simulink library "simCryogenics_lib"  (R2016a)
settings: Solver=VariableStepAuto  StartTime=0.0  StopTime=10.0  RelTol=1e-3
undefined symbols (not defined in the file or in its folder): gcbh, simscape
(part 2 of 4)

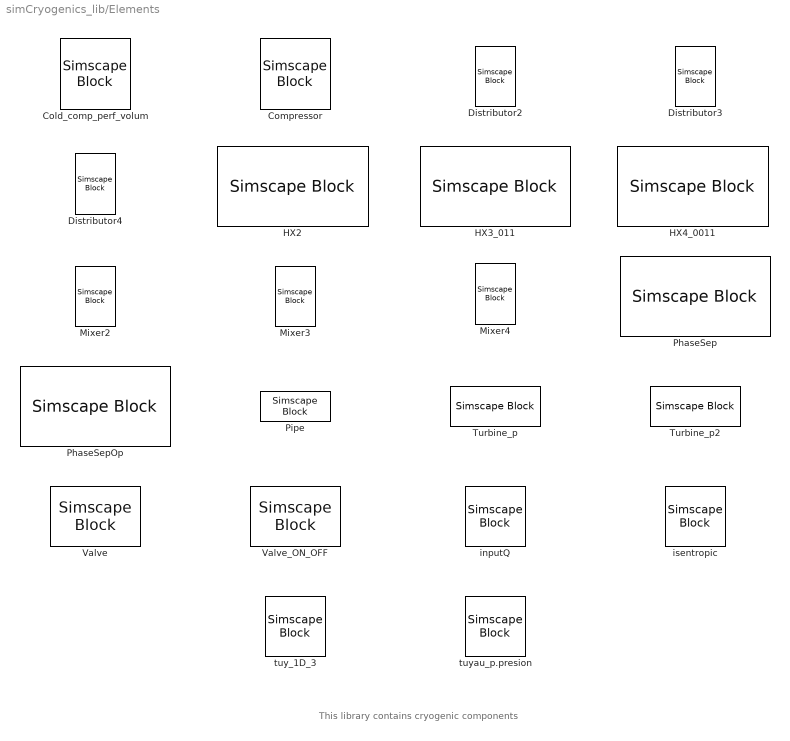
== system simCryogenics_lib/Elements ==
  note: This library contains cryogenic components
  Cold_comp_perf_volum : SimscapeBlock  DialogController=NetworkEngine.DynNeDlgSource  LoadFcn=simscape.compiler.sli.internal.callback('LoadFcn',gcbh);  SourceFile=simCryogenics.Elements.Cold_comp_perf_volum  mask(Cold_comp_perf_volum){ComponentPath=simCryogenics.Elements.Cold_comp_perf_volum, ComponentVariants=simCryogenics.Elements.Cold_comp_perf_volum, ComponentVariantNames=Cold_comp_perf_volum, ClassName=Cold_comp_perf_volum, SchemaVersion=1, rho0=1, rho0_unit=kg/m^3, rho0_conf=compiletime, eta=0.9, eta_unit=1, eta_conf=compiletime, vol=1, vol_unit=1, vol_conf=compiletime, Sin_specify=off, Sin_priority=None, Sin=0, Sin_unit=kJ/kg, HoutIs_specify=off, HoutIs_priority=None, HoutIs=0, HoutIs_unit=kJ/kg, rho_specify=off, rho_priority=None, rho=1, rho_unit=kg/m^3}
      mask prompts: rho0 "Nominal inlet density"; eta "Nominal efficiency"; vol "Volumetric"; Sin_specify "Sin"; Sin_priority "Sin"; HoutIs_specify "HoutIs"; HoutIs_priority "HoutIs"; rho_specify "rho"; rho_priority "rho"
      mask help:
      | This component is a perfect Cold Compressor with constant isentropic efficiency. It impose the flowrate on both its inlet and oulet port. The outlet port also impose the enthalpy.
      |
      | To ensure model compilation, this component inlet port must be connected to a component node that impose both enthalpy and pressure. The oulet port must be connected to a component node that impose pressure.
      |
      | The parameter eta must be in the [0 1] interval.
      mask init:
      | simscape.compiler.sli.internal.preinitmask(gcb);
      settings: CopyFcn=simscape.compiler.sli.internal.callback('CopyFcn',gcbh);  DeleteFcn=simscape.compiler.sli.internal.callback('DeleteFcn',gcbh);  ModelCloseFcn=simscape.compiler.sli.internal.callback('ModelCloseFcn',gcbh);  PreSaveFcn=simscape.compiler.sli.internal.callback('PreSaveFcn',gcbh);  PostSaveFcn=simscape.compiler.sli.internal.callback('PostSaveFcn',gcbh);  PreCopyFcn=simscape.compiler.sli.internal.callback('PreCopyFcn',gcbh);  PreDeleteFcn=simscape.compiler.sli.internal.callback('PreDeleteFcn',gcbh);
      mask Help: web(nesl_help(gcbh))
      mask TypeOptions rho0_conf: compiletime | runtime
      mask TypeOptions eta_conf: compiletime | runtime
      mask TypeOptions vol_conf: compiletime | runtime
      mask TypeOptions Sin_priority: None | Low | High
      mask TypeOptions HoutIs_priority: None | Low | High
      mask TypeOptions rho_priority: None | Low | High
      mask Display:
      | color('red');
      | port_label('LConn', 2,'M');
      | port_label('RConn', 1,'out');
      | port_label('LConn', 1,'in');
  Compressor : SimscapeBlock  DialogController=NetworkEngine.DynNeDlgSource  LoadFcn=simscape.compiler.sli.internal.callback('LoadFcn',gcbh);  SourceFile=simCryogenics.Elements.Compressor  mask(Compressor){ComponentPath=simCryogenics.Elements.Compressor, ComponentVariants=simCryogenics.Elements.Compressor, ComponentVariantNames=Compressor, ClassName=Compressor, SchemaVersion=1, Kc=0.0014, Kc_unit=kg/s/Hz/bar, Kc_conf=compiletime, lin_v=0, lin_v_unit=1, lin_v_conf=compiletime, vol=1, vol_unit=1, vol_conf=compiletime, Pnom=1, Pnom_unit=bar, Pnom_conf=compiletime, ControlInputMin=25, ControlInputMin_unit=Hz, ControlInputMin_conf=compiletime, ControlInputMax=60, ControlInputMax_unit=Hz, ControlInputMax_conf=compiletime, T_specify=off, T_priority=None, T=0, T_unit=K}
      mask prompts: Kc "Compressor constant"; lin_v "Treat input as flowrate"; vol "If flowrate input"; Pnom "Nom. press. if volumetric"; ControlInputMin "Minimum speed"; ControlInputMax "Maximum speed"; T_specify "T"; T_priority "T"
      mask help:
      | This component is an isothermal screw compressor. This component is imposing both inlet and outlet flowrate, as well as outlet temperature.
      |
      | To ensure compilation, you must connect the inlet port to a component node that impose both pressure and enthalpy (such a pipe outlet).The outlet port must be connected to a component node that impose pressure (such a pipe inlet)
      |
      | The parameter Kc must be positive
      mask init:
      | simscape.compiler.sli.internal.preinitmask(gcb);
      settings: CopyFcn=simscape.compiler.sli.internal.callback('CopyFcn',gcbh);  DeleteFcn=simscape.compiler.sli.internal.callback('DeleteFcn',gcbh);  ModelCloseFcn=simscape.compiler.sli.internal.callback('ModelCloseFcn',gcbh);  PreSaveFcn=simscape.compiler.sli.internal.callback('PreSaveFcn',gcbh);  PostSaveFcn=simscape.compiler.sli.internal.callback('PostSaveFcn',gcbh);  PreCopyFcn=simscape.compiler.sli.internal.callback('PreCopyFcn',gcbh);  PreDeleteFcn=simscape.compiler.sli.internal.callback('PreDeleteFcn',gcbh);
      mask Help: web(nesl_help(gcbh))
      mask TypeOptions Kc_conf: compiletime
      mask TypeOptions lin_v_conf: compiletime | runtime
      mask TypeOptions vol_conf: compiletime | runtime
      mask TypeOptions Pnom_conf: compiletime | runtime
      mask TypeOptions ControlInputMin_conf: compiletime | runtime
      mask TypeOptions ControlInputMax_conf: compiletime | runtime
      mask TypeOptions T_priority: None | Low | High
      mask Display:
      | color('red');
      | port_label('RConn', 1,'out');
      | port_label('LConn', 2,'in');
      | port_label('LConn', 1,'N');
  Distributor2 : SimscapeBlock  DialogController=NetworkEngine.DynNeDlgSource  LoadFcn=simscape.compiler.sli.internal.callback('LoadFcn',gcbh);  SourceFile=simCryogenics.Elements.Distributor2  mask(Distributor2){ComponentPath=simCryogenics.Elements.Distributor2, ComponentVariants=simCryogenics.Elements.Distributor2, ComponentVariantNames=Distributor2, ClassName=Distributor2, SchemaVersion=1}
      mask help:
      | This component is a distributor. It allows the user to connect one component to serval others.
      |
      | This component impose both enthalpy and pressure on its outlets and the flow rate on the inlet. To ensure compilation, the distributor inlet must be connected to a component node that impose both pressure and enthalpy (such as a pipe outlet). Every outlets must be connected to a component node that impose the flowrate (such a valve inlet)
      mask init:
      | simscape.compiler.sli.internal.preinitmask(gcb);
      settings: CopyFcn=simscape.compiler.sli.internal.callback('CopyFcn',gcbh);  DeleteFcn=simscape.compiler.sli.internal.callback('DeleteFcn',gcbh);  ModelCloseFcn=simscape.compiler.sli.internal.callback('ModelCloseFcn',gcbh);  PreSaveFcn=simscape.compiler.sli.internal.callback('PreSaveFcn',gcbh);  PostSaveFcn=simscape.compiler.sli.internal.callback('PostSaveFcn',gcbh);  PreCopyFcn=simscape.compiler.sli.internal.callback('PreCopyFcn',gcbh);  PreDeleteFcn=simscape.compiler.sli.internal.callback('PreDeleteFcn',gcbh);
      mask Help: web(nesl_help(gcbh))
      mask Display:
      | color('red');
      | port_label('RConn', 2,'');
      | port_label('RConn', 1,'');
      | port_label('LConn', 1,'');
  Distributor3 : SimscapeBlock  DialogController=NetworkEngine.DynNeDlgSource  LoadFcn=simscape.compiler.sli.internal.callback('LoadFcn',gcbh);  SourceFile=simCryogenics.Elements.Distributor3  mask(Distributor3){ComponentPath=simCryogenics.Elements.Distributor3, ComponentVariants=simCryogenics.Elements.Distributor3, ComponentVariantNames=Distributor3, ClassName=Distributor3, SchemaVersion=1}
      mask help:
      | This component is a distributor. It allows the user to connect one component to serval others.
      |
      | This component impose both enthalpy and pressure on its outlets and the flow rate on the inlet. To ensure compilation, the distributor inlet must be connected to a component node that impose both pressure and enthalpy (such as a pipe outlet). Every outlets must be connected to a component node that impose the flowrate (such a valve inlet).
      mask init:
      | simscape.compiler.sli.internal.preinitmask(gcb);
      settings: CopyFcn=simscape.compiler.sli.internal.callback('CopyFcn',gcbh);  DeleteFcn=simscape.compiler.sli.internal.callback('DeleteFcn',gcbh);  ModelCloseFcn=simscape.compiler.sli.internal.callback('ModelCloseFcn',gcbh);  PreSaveFcn=simscape.compiler.sli.internal.callback('PreSaveFcn',gcbh);  PostSaveFcn=simscape.compiler.sli.internal.callback('PostSaveFcn',gcbh);  PreCopyFcn=simscape.compiler.sli.internal.callback('PreCopyFcn',gcbh);  PreDeleteFcn=simscape.compiler.sli.internal.callback('PreDeleteFcn',gcbh);
      mask Help: web(nesl_help(gcbh))
      mask Display:
      | color('red');
      | port_label('RConn', 3,'');
      | port_label('RConn', 2,'');
      | port_label('RConn', 1,'');
      | port_label('LConn', 1,'');
  Distributor4 : SimscapeBlock  DialogController=NetworkEngine.DynNeDlgSource  LoadFcn=simscape.compiler.sli.internal.callback('LoadFcn',gcbh);  SourceFile=simCryogenics.Elements.Distributor4  mask(Distributor4){ComponentPath=simCryogenics.Elements.Distributor4, ComponentVariants=simCryogenics.Elements.Distributor4, ComponentVariantNames=Distributor4, ClassName=Distributor4, SchemaVersion=1}
      mask help:
      | This component is a distributor. It allows the user to connect one component to serval others.
      |
      | This component impose both enthalpy and pressure on its outlets and the flow rate on the inlet. To ensure compilation, the distributor inlet must be connected to a component node that impose both pressure and enthalpy (such as a pipe outlet). Every outlets must be connected to a component node that impose the flowrate (such a valve inlet).
      mask init:
      | simscape.compiler.sli.internal.preinitmask(gcb);
      settings: CopyFcn=simscape.compiler.sli.internal.callback('CopyFcn',gcbh);  DeleteFcn=simscape.compiler.sli.internal.callback('DeleteFcn',gcbh);  ModelCloseFcn=simscape.compiler.sli.internal.callback('ModelCloseFcn',gcbh);  PreSaveFcn=simscape.compiler.sli.internal.callback('PreSaveFcn',gcbh);  PostSaveFcn=simscape.compiler.sli.internal.callback('PostSaveFcn',gcbh);  PreCopyFcn=simscape.compiler.sli.internal.callback('PreCopyFcn',gcbh);  PreDeleteFcn=simscape.compiler.sli.internal.callback('PreDeleteFcn',gcbh);
      mask Help: web(nesl_help(gcbh))
      mask Display:
      | color('red');
      | port_label('RConn', 4,'');
      | port_label('RConn', 3,'');
      | port_label('RConn', 2,'');
      | port_label('RConn', 1,'');
      | port_label('LConn', 1,'');
  HX2 : SimscapeBlock  DialogController=NetworkEngine.DynNeDlgSource  LoadFcn=simscape.compiler.sli.internal.callback('LoadFcn',gcbh);  SourceFile=simCryogenics.Elements.HeatEx2  mask(HX2){ComponentPath=simCryogenics.Elements.HeatEx2, ComponentVariants=simCryogenics.Elements.HeatEx2, ComponentVariantNames=HeatEx2, ClassName=HeatEx2, SchemaVersion=1, N=6, N_unit=1, N_conf=compiletime, Vh=2.3e-3, Vh_unit=m^3, Vh_conf=compiletime, Vc=2.3e-3, Vc_unit=m^3, Vc_conf=compiletime, M=13, M_unit=kg, M_conf=compiletime, Kh=0.6, Kh_unit=s*bar/kg, Kh_conf=compiletime, Kc=0.35, Kc_unit=s*bar/kg, Kc_conf=compiletime, h=480, h_unit=J/s/K, h_conf=compiletime, Th0=10, Th0_unit=K, Th0_conf=compiletime, Ph0=16, Ph0_unit=bar, Ph0_conf=compiletime, Mh0=0.037, Mh0_unit=kg/s, Mh0_conf=compiletime, Tc0=4.5, Tc0_unit=K, Tc0_conf=compiletime, Pc0=1.1, Pc0_unit=bar, Pc0_conf=compiletime, Mc0=0.037, Mc0_unit=kg/s, Mc0_conf=compiletime}
      mask prompts: N "Number of discrete elements"; Vh "First passage volume"; Vc "Sec. passage volume"; M "Heat exchanger mass"; Kh "First passage press. drop coeff."; Kc "Sec. passage press. drop coeff."; h "Exchange coefficient"; Th0 "Initial in1 temperature"; Ph0 "Initial in1 pressure"; Mh0 "Initial out1 flowrate"; Tc0 "Initial in2 temperature"; Pc0 "Initial out2 pressure"; Mc0 "Initial in2 flowrate"
      mask help:
      | This component is a two branches cross-current heat Exchanger
      |
      | The following variables are imposed to others components: - in1 node : flow rate - out1 node : pressure and enthalpy - in2 node : enthalpy and flow rate - out2 node : pressure
      |
      | To ensure compilation, the heat Exchanger must be connected to components nodes that impose: - pressure and enthalpy on the in1 node - flowrate on the out1 node - flowrate and enthalpy on the in2 node - pressure on the out2 node
      |
      | Note : the initial temperature/flowrate/presure conditions should be equal to the actual value on the scheme (especially for heat exchangers connected to sources).
      |
      | All parameters must be positive
      mask init:
      | simscape.compiler.sli.internal.preinitmask(gcb);
      settings: CopyFcn=simscape.compiler.sli.internal.callback('CopyFcn',gcbh);  DeleteFcn=simscape.compiler.sli.internal.callback('DeleteFcn',gcbh);  ModelCloseFcn=simscape.compiler.sli.internal.callback('ModelCloseFcn',gcbh);  PreSaveFcn=simscape.compiler.sli.internal.callback('PreSaveFcn',gcbh);  PostSaveFcn=simscape.compiler.sli.internal.callback('PostSaveFcn',gcbh);  PreCopyFcn=simscape.compiler.sli.internal.callback('PreCopyFcn',gcbh);  PreDeleteFcn=simscape.compiler.sli.internal.callback('PreDeleteFcn',gcbh);
      mask Help: web(nesl_help(gcbh))
      mask TypeOptions N_conf: compiletime
      mask TypeOptions Vh_conf: compiletime
      mask TypeOptions Vc_conf: compiletime
      mask TypeOptions M_conf: compiletime
      mask TypeOptions Kh_conf: compiletime
      mask TypeOptions Kc_conf: compiletime
      mask TypeOptions h_conf: compiletime
      mask TypeOptions Th0_conf: compiletime
      mask TypeOptions Ph0_conf: compiletime
      mask TypeOptions Mh0_conf: compiletime
      mask TypeOptions Tc0_conf: compiletime
      mask TypeOptions Pc0_conf: compiletime
      mask TypeOptions Mc0_conf: compiletime
      mask Display:
      | color('red');
      | port_label('RConn', 2,'out1');
      | port_label('RConn', 1,'in2');
      | port_label('LConn', 2,'in1');
      | port_label('LConn', 1,'out2');
  HX3_011 : SimscapeBlock  DialogController=NetworkEngine.DynNeDlgSource  LoadFcn=simscape.compiler.sli.internal.callback('LoadFcn',gcbh);  SourceFile=simCryogenics.Elements.HeatEx3_011  mask(HX3_011){ComponentPath=simCryogenics.Elements.HeatEx3_011, ComponentVariants=simCryogenics.Elements.HeatEx3_011, ComponentVariantNames=HeatEx3_011, ClassName=HeatEx3_011, SchemaVersion=1, N=8, N_unit=1, N_conf=compiletime, Vh=2.3e-3, Vh_unit=m^3, Vh_conf=compiletime, Vm=2.3e-3, Vm_unit=m^3, Vm_conf=compiletime, Vc=2.3e-3, Vc_unit=m^3, Vc_conf=compiletime, M=13, M_unit=kg, M_conf=compiletime, Kh=0, Kh_unit=s*bar/kg, Kh_conf=compiletime, Km=0, Km_unit=s*bar/kg, Km_conf=compiletime, Kc=0, Kc_unit=s*bar/kg, Kc_conf=compiletime, hh_m=400, hh_m_unit=J/s/K, hh_m_conf=compiletime, hh_c=400, hh_c_unit=J/s/K, hh_c_conf=compiletime, hm_c=400, hm_c_unit=J/s/K, hm_c_conf=compiletime, Th0=10, Th0_unit=K, Th0_conf=compiletime, Ph0=16, Ph0_unit=bar, Ph0_conf=compiletime, Mh0=0.037, Mh0_unit=kg/s, Mh0_conf=compiletime, Tm0=4.5, Tm0_unit=K, Tm0_conf=compiletime, Pm0=1.1, Pm0_unit=bar, Pm0_conf=compiletime, Mm0=0.037, Mm0_unit=kg/s, Mm0_conf=compiletime, Tc0=4.5, Tc0_unit=K, Tc0_conf=compiletime, Pc0=1.1, Pc0_unit=bar, Pc0_conf=compiletime, Mc0=0.037, Mc0_unit=kg/s, Mc0_conf=compiletime, sensh=0, sensh_unit=1, sensh_conf=compiletime, sensm=1, sensm_unit=1, sensm_conf=compiletime, sensc=1, sensc_unit=1, sensc_conf=compiletime}
      mask prompts: N "Number of discrete elements"; Vh "First passage volume"; Vm "Second passage volume"; Vc "Third passage volume"; M "Heat exchanger mass"; Kh "First passage pressure drop"; Km "Second passage pressure drop"; Kc "Third passage pressure drop"; hh_m "Ex. coeff. between pass. 1 and 2"; hh_c "Ex. coeff. between pass. 1 and 3"; hm_c "Ex. coeff. between pass. 2 and 3"; Th0 "Initial in1 temperature"; Ph0 "Initial in1 pressure"; Mh0 "Initial out1 flowrate"; Tm0 "Initial in2 temperature"; Pm0 "Initial out2 pressure"; Mm0 "Initial in2 flowrate"; Tc0 "Initial in3 temperature"; Pc0 "Initial out3 pressure"; Mc0 "Initial in3 flowrate"; sensh "Sens hot flow"; sensm "Sens middle flow"; sensc "Sens cold flow"
      mask help:
      | This component is a three branches cross-current heat Exchanger
      |
      | The following variables are imposed to others components: - in1 node : pressure and enthalpy - out1 node :  flow rate - in2/3 node : enthalpy and flow rate - out2/3 node : pressure
      |
      | To ensure compilation, the heat Exchanger must be connected to components nodes that impose: - pressure and enthalpy on the in1 node - flowrate on the out1 node - flowrate and enthalpy on the in2/3 node - pressure on the out2/3 node
      |
      | Note : the initial temperature/flowrate/presure conditions should be equal to the actual value on the scheme (especially for heat exchangers connected to sources).
      |
      | All parameters must be positive
      mask init:
      | simscape.compiler.sli.internal.preinitmask(gcb);
      settings: CopyFcn=simscape.compiler.sli.internal.callback('CopyFcn',gcbh);  DeleteFcn=simscape.compiler.sli.internal.callback('DeleteFcn',gcbh);  ModelCloseFcn=simscape.compiler.sli.internal.callback('ModelCloseFcn',gcbh);  PreSaveFcn=simscape.compiler.sli.internal.callback('PreSaveFcn',gcbh);  PostSaveFcn=simscape.compiler.sli.internal.callback('PostSaveFcn',gcbh);  PreCopyFcn=simscape.compiler.sli.internal.callback('PreCopyFcn',gcbh);  PreDeleteFcn=simscape.compiler.sli.internal.callback('PreDeleteFcn',gcbh);
      mask Help: web(nesl_help(gcbh))
      mask TypeOptions N_conf: compiletime
      mask TypeOptions Vh_conf: compiletime
      mask TypeOptions Vm_conf: compiletime
      mask TypeOptions Vc_conf: compiletime
      mask TypeOptions M_conf: compiletime
      mask TypeOptions Kh_conf: compiletime
      mask TypeOptions Km_conf: compiletime
      mask TypeOptions Kc_conf: compiletime
      mask TypeOptions hh_m_conf: compiletime
      mask TypeOptions hh_c_conf: compiletime
      mask TypeOptions hm_c_conf: compiletime
      mask TypeOptions Th0_conf: compiletime
      mask TypeOptions Ph0_conf: compiletime
      mask TypeOptions Mh0_conf: compiletime
      mask TypeOptions Tm0_conf: compiletime
      mask TypeOptions Pm0_conf: compiletime
      mask TypeOptions Mm0_conf: compiletime
      mask TypeOptions Tc0_conf: compiletime
      mask TypeOptions Pc0_conf: compiletime
      mask TypeOptions Mc0_conf: compiletime
      mask TypeOptions sensh_conf: compiletime
      mask TypeOptions sensm_conf: compiletime
      mask TypeOptions sensc_conf: compiletime
      mask Display:
      | color('red');
      | port_label('LConn', 3,'in1');
      | port_label('LConn', 2,'out2');
      | port_label('LConn', 1,'out3');
      | port_label('RConn', 3,'out1');
      | port_label('RConn', 2,'in2');
      | port_label('RConn', 1,'in3');
  HX4_0011 : SimscapeBlock  DialogController=NetworkEngine.DynNeDlgSource  LoadFcn=simscape.compiler.sli.internal.callback('LoadFcn',gcbh);  SourceFile=simCryogenics.Elements.HeatEx4_0011  mask(HX4_0011){ComponentPath=simCryogenics.Elements.HeatEx4_0011, ComponentVariants=simCryogenics.Elements.HeatEx4_0011, ComponentVariantNames=HeatEx4_0011, ClassName=HeatEx4_0011, SchemaVersion=1, N=8, N_unit=1, N_conf=compiletime, Vh=2.3e-3, Vh_unit=m^3, Vh_conf=compiletime, Vm=2.3e-3, Vm_unit=m^3, Vm_conf=compiletime, Vc=2.3e-3, Vc_unit=m^3, Vc_conf=compiletime, Vvc=2.3e-3, Vvc_unit=m^3, Vvc_conf=compiletime, M=13, M_unit=kg, M_conf=compiletime, Kh=0, Kh_unit=s*bar/kg, Kh_conf=compiletime, Km=0, Km_unit=s*bar/kg, Km_conf=compiletime, Kc=0, Kc_unit=s*bar/kg, Kc_conf=compiletime, Kvc=0, Kvc_unit=s*bar/kg, Kvc_conf=compiletime, hh_m=800, hh_m_unit=J/s/K, hh_m_conf=compiletime, hh_c=800, hh_c_unit=J/s/K, hh_c_conf=compiletime, hh_vc=800, hh_vc_unit=J/s/K, hh_vc_conf=compiletime, hm_c=800, hm_c_unit=J/s/K, hm_c_conf=compiletime, hm_vc=800, hm_vc_unit=J/s/K, hm_vc_conf=compiletime, hc_vc=800, hc_vc_unit=J/s/K, hc_vc_conf=compiletime, Th0=10, Th0_unit=K, Th0_conf=compiletime, Ph0=16, Ph0_unit=bar, Ph0_conf=compiletime, Mh0=0.037, Mh0_unit=kg/s, Mh0_conf=compiletime, Tm0=4.5, Tm0_unit=K, Tm0_conf=compiletime, Pm0=1.1, Pm0_unit=bar, Pm0_conf=compiletime, Mm0=0.037, Mm0_unit=kg/s, Mm0_conf=compiletime, Tc0=4.5, Tc0_unit=K, Tc0_conf=compiletime, Pc0=1.1, Pc0_unit=bar, Pc0_conf=compiletime, Mc0=0.037, Mc0_unit=kg/s, Mc0_conf=compiletime, Tvc0=4.5, Tvc0_unit=K, Tvc0_conf=compiletime, Pvc0=1.1, Pvc0_unit=bar, Pvc0_conf=compiletime, Mvc0=0.037, Mvc0_unit=kg/s, Mvc0_conf=compiletime, sensh=0, sensh_unit=1, sensh_conf=compiletime, sensm=0, sensm_unit=1, sensm_conf=compiletime, sensc=1, sensc_unit=1, sensc_conf=compiletime, sensvc=1, sensvc_unit=1, sensvc_conf=compiletime}
      mask prompts: N "Number of discrete elements"; Vh "First passage volume"; Vm "Second passage volume"; Vc "Third passage volume"; Vvc "Fourth passage volume"; M "Heat exchanger mass"; Kh "First passage pressure drop"; Km "Second passage pressure drop"; Kc "Third passage pressure drop"; Kvc "Fourth passage pressure drop"; hh_m "Ex. coeff. between pass. 1 and 2"; hh_c "Ex. coeff. between pass. 1 and 3"; hh_vc "Ex. coeff. between pass. 1 and 4"; hm_c "Ex. coeff. between pass. 2 and 3"; hm_vc "Ex. coeff. between pass. 2 and 4"; hc_vc "Ex. coeff. between pass. 3 and 4"; Th0 "Initial in1 temperature"; Ph0 "Initial in1 pressure"; Mh0 "Initial out1 flowrate"; Tm0 "Initial in2 temperature"; Pm0 "Initial out2 pressure"; Mm0 "Initial in2 flowrate"; Tc0 "Initial in3 temperature"; Pc0 "Initial out3 pressure"; Mc0 "Initial in3 flowrate"; Tvc0 "Initial in4 temperature"; Pvc0 "Initial out4 pressure"; Mvc0 "Initial in4 flowrate"; sensh "Sens hot  flow"; sensm "Sens middle flow"; sensc "Sens cold flow"; sensvc "Sens very cold flow"
      mask help:
      | This component is a three branches cross-current heat Exchanger
      |
      | The following variables are imposed to others components: - in1/2 node : pressure and enthalpy - out1/2 node : flow rate - in3/4 node : enthalpy and flow rate - out3/4 node : pressure
      |
      | To ensure compilation, the heat Exchanger must be connected to components nodes that impose: - pressure and enthalpy on the in1/2 node - flowrate on the out1/2 node - flowrate and enthalpy on the in3/4 node - pressure on the out3/4 node
      |
      | Note : the initial temperature/flowrate/presure conditions should be equal to the actual value on the scheme (especially for heat exchangers connected to sources).
      |
      | All parameters must be positive
      mask init:
      | simscape.compiler.sli.internal.preinitmask(gcb);
      settings: CopyFcn=simscape.compiler.sli.internal.callback('CopyFcn',gcbh);  DeleteFcn=simscape.compiler.sli.internal.callback('DeleteFcn',gcbh);  ModelCloseFcn=simscape.compiler.sli.internal.callback('ModelCloseFcn',gcbh);  PreSaveFcn=simscape.compiler.sli.internal.callback('PreSaveFcn',gcbh);  PostSaveFcn=simscape.compiler.sli.internal.callback('PostSaveFcn',gcbh);  PreCopyFcn=simscape.compiler.sli.internal.callback('PreCopyFcn',gcbh);  PreDeleteFcn=simscape.compiler.sli.internal.callback('PreDeleteFcn',gcbh);
      mask Help: web(nesl_help(gcbh))
      mask TypeOptions N_conf: compiletime
      mask TypeOptions Vh_conf: compiletime
      mask TypeOptions Vm_conf: compiletime
      mask TypeOptions Vc_conf: compiletime
      mask TypeOptions Vvc_conf: compiletime
      mask TypeOptions M_conf: compiletime
      mask TypeOptions Kh_conf: compiletime
      mask TypeOptions Km_conf: compiletime
      mask TypeOptions Kc_conf: compiletime
      mask TypeOptions Kvc_conf: compiletime | runtime
      mask TypeOptions hh_m_conf: compiletime
      mask TypeOptions hh_c_conf: compiletime
      mask TypeOptions hh_vc_conf: compiletime
      mask TypeOptions hm_c_conf: compiletime
      mask TypeOptions hm_vc_conf: compiletime
      mask TypeOptions hc_vc_conf: compiletime
      mask TypeOptions Th0_conf: compiletime
      mask TypeOptions Ph0_conf: compiletime
      mask TypeOptions Mh0_conf: compiletime
      mask TypeOptions Tm0_conf: compiletime
      mask TypeOptions Pm0_conf: compiletime
      mask TypeOptions Mm0_conf: compiletime
      mask TypeOptions Tc0_conf: compiletime
      mask TypeOptions Pc0_conf: compiletime
      mask TypeOptions Mc0_conf: compiletime
      mask TypeOptions Tvc0_conf: compiletime
      mask TypeOptions Pvc0_conf: compiletime
      mask TypeOptions Mvc0_conf: compiletime
      mask TypeOptions sensh_conf: compiletime
      mask TypeOptions sensm_conf: compiletime
      mask TypeOptions sensc_conf: compiletime
      mask TypeOptions sensvc_conf: compiletime
      mask Display:
      | color('red');
      | port_label('LConn', 4,'in1');
      | port_label('LConn', 3,'in2');
      | port_label('LConn', 2,'out3');
      | port_label('LConn', 1,'out4');
      | port_label('RConn', 4,'out1');
      | port_label('RConn', 3,'out2');
      | port_label('RConn', 2,'in3');
      | port_label('RConn', 1,'in4');
  Mixer2 : SimscapeBlock  DialogController=NetworkEngine.DynNeDlgSource  LoadFcn=simscape.compiler.sli.internal.callback('LoadFcn',gcbh);  SourceFile=simCryogenics.Elements.Mixer2  mask(Mixer2){ComponentPath=simCryogenics.Elements.Mixer2, ComponentVariants=simCryogenics.Elements.Mixer2, ComponentVariantNames=Mixer2, ClassName=Mixer2, SchemaVersion=1}
      mask help:
      | This component is a mixer. It allows to connect several components to another one.
      |
      | This component impose both enthalpy and flowrate on the outlet and pressure on inlets. To ensure compilation, the mixer inlets must be connected to a component node that impose pressure (such as a pipe inlet). The outlet must be connected to a component node that impose both flowrate and enthalpy (such a valve outlet)
      mask init:
      | simscape.compiler.sli.internal.preinitmask(gcb);
      settings: CopyFcn=simscape.compiler.sli.internal.callback('CopyFcn',gcbh);  DeleteFcn=simscape.compiler.sli.internal.callback('DeleteFcn',gcbh);  ModelCloseFcn=simscape.compiler.sli.internal.callback('ModelCloseFcn',gcbh);  PreSaveFcn=simscape.compiler.sli.internal.callback('PreSaveFcn',gcbh);  PostSaveFcn=simscape.compiler.sli.internal.callback('PostSaveFcn',gcbh);  PreCopyFcn=simscape.compiler.sli.internal.callback('PreCopyFcn',gcbh);  PreDeleteFcn=simscape.compiler.sli.internal.callback('PreDeleteFcn',gcbh);
      mask Help: web(nesl_help(gcbh))
      mask Display:
      | color('red');
      | port_label('RConn', 1,'');
      | port_label('LConn', 2,'');
      | port_label('LConn', 1,'');
  Mixer3 : SimscapeBlock  DialogController=NetworkEngine.DynNeDlgSource  LoadFcn=simscape.compiler.sli.internal.callback('LoadFcn',gcbh);  SourceFile=simCryogenics.Elements.Mixer3  mask(Mixer3){ComponentPath=simCryogenics.Elements.Mixer3, ComponentVariants=simCryogenics.Elements.Mixer3, ComponentVariantNames=Mixer3, ClassName=Mixer3, SchemaVersion=1}
      mask help:
      | This component is a mixer. It allows to connect several components to another one.
      |
      | This component impose both enthalpy and flowrate on the outlet and pressure on inlets. To ensure compilation, the mixer inlets must be connected to a component node that impose pressure (such as a pipe inlet). The outlet must be connected to a component node that impose both flowrate and enthalpy (such a valve outlet)
      mask init:
      | simscape.compiler.sli.internal.preinitmask(gcb);
      settings: CopyFcn=simscape.compiler.sli.internal.callback('CopyFcn',gcbh);  DeleteFcn=simscape.compiler.sli.internal.callback('DeleteFcn',gcbh);  ModelCloseFcn=simscape.compiler.sli.internal.callback('ModelCloseFcn',gcbh);  PreSaveFcn=simscape.compiler.sli.internal.callback('PreSaveFcn',gcbh);  PostSaveFcn=simscape.compiler.sli.internal.callback('PostSaveFcn',gcbh);  PreCopyFcn=simscape.compiler.sli.internal.callback('PreCopyFcn',gcbh);  PreDeleteFcn=simscape.compiler.sli.internal.callback('PreDeleteFcn',gcbh);
      mask Help: web(nesl_help(gcbh))
      mask Display:
      | color('red');
      | port_label('LConn', 3,'');
      | port_label('RConn', 1,'');
      | port_label('LConn', 2,'');
      | port_label('LConn', 1,'');
  Mixer4 : SimscapeBlock  DialogController=NetworkEngine.DynNeDlgSource  LoadFcn=simscape.compiler.sli.internal.callback('LoadFcn',gcbh);  SourceFile=simCryogenics.Elements.Mixer4  mask(Mixer4){ComponentPath=simCryogenics.Elements.Mixer4, ComponentVariants=simCryogenics.Elements.Mixer4, ComponentVariantNames=Mixer4, ClassName=Mixer4, SchemaVersion=1}
      mask help:
      | This component is a mixer. It allows to connect several components to another one.
      |
      | This component impose both enthalpy and flowrate on the outlet and pressure on inlets. To ensure compilation, the mixer inlets must be connected to a component node that impose pressure (such as a pipe inlet). The outlet must be connected to a component node that impose both flowrate and enthalpy (such a valve outlet)
      mask init:
      | simscape.compiler.sli.internal.preinitmask(gcb);
      settings: CopyFcn=simscape.compiler.sli.internal.callback('CopyFcn',gcbh);  DeleteFcn=simscape.compiler.sli.internal.callback('DeleteFcn',gcbh);  ModelCloseFcn=simscape.compiler.sli.internal.callback('ModelCloseFcn',gcbh);  PreSaveFcn=simscape.compiler.sli.internal.callback('PreSaveFcn',gcbh);  PostSaveFcn=simscape.compiler.sli.internal.callback('PostSaveFcn',gcbh);  PreCopyFcn=simscape.compiler.sli.internal.callback('PreCopyFcn',gcbh);  PreDeleteFcn=simscape.compiler.sli.internal.callback('PreDeleteFcn',gcbh);
      mask Help: web(nesl_help(gcbh))
      mask Display:
      | color('red');
      | port_label('LConn', 4,'');
      | port_label('LConn', 3,'');
      | port_label('RConn', 1,'');
      | port_label('LConn', 2,'');
      | port_label('LConn', 1,'');
  PhaseSep : SimscapeBlock  DialogController=NetworkEngine.DynNeDlgSource  LoadFcn=simscape.compiler.sli.internal.callback('LoadFcn',gcbh);  SourceFile=simCryogenics.Elements.PhaseSep  mask(PhaseSep){ComponentPath=simCryogenics.Elements.PhaseSep, ComponentVariants=simCryogenics.Elements.PhaseSep, ComponentVariantNames=PhaseSep, ClassName=PhaseSep, SchemaVersion=1, Ideal1=1, Ideal1_unit=1, Ideal1_conf=compiletime, DeltaT1=0.05, DeltaT1_unit=K, DeltaT1_conf=compiletime, N1=10, N1_unit=1, N1_conf=compiletime, h1=400, h1_unit=W/K, h1_conf=compiletime, Ideal2=1, Ideal2_unit=1, Ideal2_conf=compiletime, DeltaT2=0.05, DeltaT2_unit=K, DeltaT2_conf=compiletime, N2=10, N2_unit=1, N2_conf=compiletime, h2=400, h2_unit=W/K, h2_conf=compiletime, hmax=1.5, hmax_unit=m, hmax_conf=compiletime, S=0.2, S_unit=m^2, S_conf=compiletime, P0=1.2, P0_unit=bar, P0_conf=compiletime, h0=50, h0_unit=1, h0_conf=compiletime, T0=4.5, T0_unit=K, T0_conf=compiletime}
      mask prompts: Ideal1 "Ideal 1/0"; DeltaT1 "Delta T"; N1 "Number of discrete elements"; h1 "Exchange coefficient"; Ideal2 "Ideal : 0/1"; DeltaT2 "Delta T"; N2 "Number of discrete elements"; h2 "Exchange coefficient"; hmax "Bath height"; S "Surface"; P0 "Initial pressure"; h0 "Initial liquid height"; T0 "Initial bath temperature"
      mask help:
      | This component is a phase separator including two heat exchangers.
      |
      | About the phase separator: Ports marked as outlets are imposing impose both pressure and enthalpy and must be connected to a component node that impose flowrate to ensure compilation. Port marked as inlet are imposing pressure and must be connected to a component node that impose both enthalpy and flow rate (such as a valve outlet).
      |
      | About the heat exchangers: inlets ports impose flowrate and must be connected to a component port that impose both enthalpy and pressure. Outlets ports impose both enthalpy and pressure and must be connected to a component port that impose the flowrate.
      |
      | All parameters must be positive.
      mask init:
      | simscape.compiler.sli.internal.preinitmask(gcb);
      settings: CopyFcn=simscape.compiler.sli.internal.callback('CopyFcn',gcbh);  DeleteFcn=simscape.compiler.sli.internal.callback('DeleteFcn',gcbh);  ModelCloseFcn=simscape.compiler.sli.internal.callback('ModelCloseFcn',gcbh);  PreSaveFcn=simscape.compiler.sli.internal.callback('PreSaveFcn',gcbh);  PostSaveFcn=simscape.compiler.sli.internal.callback('PostSaveFcn',gcbh);  PreCopyFcn=simscape.compiler.sli.internal.callback('PreCopyFcn',gcbh);  PreDeleteFcn=simscape.compiler.sli.internal.callback('PreDeleteFcn',gcbh);
      mask Help: web(nesl_help(gcbh))
      mask TypeOptions Ideal1_conf: compiletime | runtime
      mask TypeOptions DeltaT1_conf: compiletime | runtime
      mask TypeOptions N1_conf: compiletime | runtime
      mask TypeOptions h1_conf: compiletime | runtime
      mask TypeOptions Ideal2_conf: compiletime | runtime
      mask TypeOptions DeltaT2_conf: compiletime | runtime
      mask TypeOptions N2_conf: compiletime | runtime
      mask TypeOptions h2_conf: compiletime | runtime
      mask TypeOptions hmax_conf: compiletime | runtime
      mask TypeOptions S_conf: compiletime | runtime
      mask TypeOptions P0_conf: compiletime
      mask TypeOptions h0_conf: compiletime
      mask TypeOptions T0_conf: compiletime
      mask Display:
      | color('red');
      | port_label('RConn', 5,'h');
      | port_label('LConn', 5,'x');
      | port_label('RConn', 4,'Q');
      | port_label('LConn', 4,'inM');
      | port_label('RConn', 3,'out2');
      | port_label('LConn', 3,'in2');
      | port_label('RConn', 2,'out1');
      | port_label('LConn', 2,'in1');
      | port_label('RConn', 1,'outL');
      | port_label('LConn', 1,'outG');
  PhaseSepOp : SimscapeBlock  DialogController=NetworkEngine.DynNeDlgSource  LoadFcn=simscape.compiler.sli.internal.callback('LoadFcn',gcbh);  SourceFile=simCryogenics.Elements.PhaseSepOp  mask(PhaseSepOp){ComponentPath=simCryogenics.Elements.PhaseSepOp, ComponentVariants=simCryogenics.Elements.PhaseSepOp, ComponentVariantNames=PhaseSepOp, ClassName=PhaseSepOp, SchemaVersion=1, Ideal1=1, Ideal1_unit=1, Ideal1_conf=compiletime, DeltaT1=0.05, DeltaT1_unit=K, DeltaT1_conf=compiletime, N1=10, N1_unit=1, N1_conf=compiletime, h1=400, h1_unit=W/K, h1_conf=compiletime, Ideal2=1, Ideal2_unit=1, Ideal2_conf=compiletime, DeltaT2=0.05, DeltaT2_unit=K, DeltaT2_conf=compiletime, N2=10, N2_unit=1, N2_conf=compiletime, h2=400, h2_unit=W/K, h2_conf=compiletime, hmax=1.5, hmax_unit=m, hmax_conf=compiletime, S=0.2, S_unit=m^2, S_conf=compiletime, h0=50, h0_unit=1, h0_conf=compiletime}
      mask prompts: Ideal1 "Ideal 1/0"; DeltaT1 "Delta T"; N1 "Number of discrete elements"; h1 "Exchange coefficient"; Ideal2 "Ideal : 0/1"; DeltaT2 "Delta T"; N2 "Number of discrete elements"; h2 "Exchange coefficient"; hmax "Bath height"; S "Surface"; h0 "Initial liquid height"
      mask help:
      | This component is an open phase separator including two heat exchangers.
      |
      | The open phase separator impose: - flowrate and enthalpy on port outG - pressure and enthalpy on port outL - pressure on port inM
      |
      | About the heat exchangers: inlets ports impose flowrate and must be connected to a component port that impose both enthalpy and pressure. Outlets ports impose both enthalpy and pressure and must be connected to a component port that impose the flowrate.
      |
      | All parameters must be positive.
      mask init:
      | simscape.compiler.sli.internal.preinitmask(gcb);
      settings: CopyFcn=simscape.compiler.sli.internal.callback('CopyFcn',gcbh);  DeleteFcn=simscape.compiler.sli.internal.callback('DeleteFcn',gcbh);  ModelCloseFcn=simscape.compiler.sli.internal.callback('ModelCloseFcn',gcbh);  PreSaveFcn=simscape.compiler.sli.internal.callback('PreSaveFcn',gcbh);  PostSaveFcn=simscape.compiler.sli.internal.callback('PostSaveFcn',gcbh);  PreCopyFcn=simscape.compiler.sli.internal.callback('PreCopyFcn',gcbh);  PreDeleteFcn=simscape.compiler.sli.internal.callback('PreDeleteFcn',gcbh);
      mask Help: web(nesl_help(gcbh))
      mask TypeOptions Ideal1_conf: compiletime | runtime
      mask TypeOptions DeltaT1_conf: compiletime | runtime
      mask TypeOptions N1_conf: compiletime | runtime
      mask TypeOptions h1_conf: compiletime | runtime
      mask TypeOptions Ideal2_conf: compiletime | runtime
      mask TypeOptions DeltaT2_conf: compiletime | runtime
      mask TypeOptions N2_conf: compiletime | runtime
      mask TypeOptions h2_conf: compiletime | runtime
      mask TypeOptions hmax_conf: compiletime | runtime
      mask TypeOptions S_conf: compiletime | runtime
      mask TypeOptions h0_conf: compiletime
      mask Display:
      | color('red');
      | port_label('RConn', 5,'h');
      | port_label('LConn', 5,'x');
      | port_label('RConn', 4,'Q');
      | port_label('LConn', 4,'inM');
      | port_label('RConn', 3,'out2');
      | port_label('LConn', 3,'in2');
      | port_label('RConn', 2,'out1');
      | port_label('LConn', 2,'in1');
      | port_label('RConn', 1,'outL');
      | port_label('LConn', 1,'outG');
  Pipe : SimscapeBlock  DialogController=NetworkEngine.DynNeDlgSource  LoadFcn=simscape.compiler.sli.internal.callback('LoadFcn',gcbh);  SourceFile=simCryogenics.Elements.Pipe  mask(Pipe){ComponentPath=simCryogenics.Elements.Pipe, ComponentVariants=simCryogenics.Elements.Pipe, ComponentVariantNames=Pipe, ClassName=Pipe, SchemaVersion=1, Vol=1, Vol_unit=m^3, Vol_conf=compiletime, Ideal=0, Ideal_unit=1, Ideal_conf=compiletime, P0=1, P0_unit=bar, P0_conf=compiletime, T0=300, T0_unit=K, T0_conf=compiletime}
      mask prompts: Vol "Pipe volume"; Ideal "Ideal 1/0"; P0 "Initial pressure"; T0 "Initial temperature"
      mask help:
      | Pipe
      |
      | This component models a 0D pipe. It differs from a simple port connection because it imposes a variable pressure on both inlet and outlet port. On the outlet port a temperature is also imposed.
      |
      | The inlet port must be connected to a port that imposes both a temperature and flow rate (such as a compressor outlet or a valve outlet).  The outlet port must be connected to a port that impose a flow rate (such as a compressor inlet or a valve inlet).
      |
      | If you want to use an ideal pipe (differentiation of pressure, P, with regard to time) the parameter 'Ideal' must be set to 1. Otherwise, a non-Ideal pipe (differentiation of rho and u with regard to time) will be used.
      |
      | The parameters Vol and initial conditions P0 and T0 must be positive
      |
      | Note :  The initial values for pressure and temperature should be set to correspond with the actual values imposed on the component at the time of initialization.
      mask init:
      | simscape.compiler.sli.internal.preinitmask(gcb);
      settings: CopyFcn=simscape.compiler.sli.internal.callback('CopyFcn',gcbh);  DeleteFcn=simscape.compiler.sli.internal.callback('DeleteFcn',gcbh);  ModelCloseFcn=simscape.compiler.sli.internal.callback('ModelCloseFcn',gcbh);  PreSaveFcn=simscape.compiler.sli.internal.callback('PreSaveFcn',gcbh);  PostSaveFcn=simscape.compiler.sli.internal.callback('PostSaveFcn',gcbh);  PreCopyFcn=simscape.compiler.sli.internal.callback('PreCopyFcn',gcbh);  PreDeleteFcn=simscape.compiler.sli.internal.callback('PreDeleteFcn',gcbh);
      mask Help: web(nesl_help(gcbh))
      mask TypeOptions Vol_conf: compiletime
      mask TypeOptions Ideal_conf: compiletime
      mask TypeOptions P0_conf: compiletime
      mask TypeOptions T0_conf: compiletime
      mask Display:
      | color('red');
      | port_label('RConn', 1,'out');
      | port_label('LConn', 1,'in');
  Turbine_p : SimscapeBlock  DialogController=NetworkEngine.DynNeDlgSource  LoadFcn=simscape.compiler.sli.internal.callback('LoadFcn',gcbh);  SourceFile=simCryogenics.Elements.Turbine_p  mask(Turbine_p){ComponentPath=simCryogenics.Elements.Turbine_p, ComponentVariants=simCryogenics.Elements.Turbine_p, ComponentVariantNames=Turbine_p, ClassName=Turbine_p, SchemaVersion=1, A=5e-6, A_unit=m^2, A_conf=compiletime, D=0.0255, D_unit=m, D_conf=compiletime, Mass=0.02, Mass_unit=kg, Mass_conf=compiletime, cst_eff=0, cst_eff_unit=1, cst_eff_conf=compiletime, eta0=0.8, eta0_unit=1, eta0_conf=compiletime, Tin0=20, Tin0_unit=K, Tin0_conf=compiletime, Pin0=16, Pin0_unit=bar, Pin0_conf=compiletime, Pout0=1.2, Pout0_unit=bar, Pout0_conf=compiletime, N0=2250, N0_unit=1/s, N0_conf=compiletime, Q0=0, Q0_unit=W, Q0_conf=compiletime, v0=0, v0_unit=1, v0_conf=compiletime, I=0, I_unit=kg*m^2, I_conf=compiletime, gamma_specify=off, gamma_priority=None, gamma=0, gamma_unit=1, C_specify=off, C_priority=None, C=0, C_unit=1, Z_specify=off, Z_priority=None, Z=0, Z_unit=1, Cp_specify=off, Cp_priority=None, Cp=0, Cp_unit=kJ/kg/K, Sin_specify=off, Sin_priority=None, Sin=0, Sin_unit=kJ/kg, T_specify=off, T_priority=None, T=0, T_unit=K, HoutIs_specify=off, HoutIs_priority=None, HoutIs=0, HoutIs_unit=kJ/kg, u1_specify=off, u1_priority=None, u1=0, u1_unit=m/s, c1_specify=off, c1_priority=None, c1=0, c1_unit=m/s, v_specify=off, v_priority=None, v=0, v_unit=1, eta_specify=off, eta_priority=None, eta=0, eta_unit=1, eta_var_specify=off, eta_var_priority=None, eta_var=0, eta_var_unit=1, N_specify=off, N_priority=None, N=0, N_unit=rad/s, Q_specify=off, Q_priority=None, Q=0, Q_unit=W}
      mask prompts: A "Section pass"; D "Blade diameter"; Mass "Shaft mass"; cst_eff "Constant efficiency"; eta0 "Nominal efficiency"; Tin0 "Nominal inlet temperature"; Pin0 "Nominal inlet pressure"; Pout0 "Nominal outlet pressure"; N0 "Nominal speed"; v0 "velocities ratio"; gamma_specify "gamma"; gamma_priority "gamma"; C_specify "C"; C_priority "C"; Z_specify "Z"; Z_priority "Z"; Cp_specify "Cp"; Cp_priority "Cp"; Sin_specify "Sin"; Sin_priority "Sin"; T_specify "T"; T_priority "T"; HoutIs_specify "HoutIs"; HoutIs_priority "HoutIs"; u1_specify "u1"; u1_priority "u1"; c1_specify "c1"; c1_priority "c1"; v_specify "v"; v_priority "v"; eta_specify "eta"; eta_priority "eta"; eta_var_specify "eta_var"; eta_var_priority "eta_var"; N_specify "N"; N_priority "N"; Q_specify "Q"; Q_priority "Q"
      mask help:
      | This component is a cryogenic Turbine with constant or variable isentropic efficiency. It impose the flowrate on both its inlet and oulet port. The outlet port also impose the temperature.
      |
      | To ensure compilation, this component inlet port must be connected to a component port that impose both temperature and pressure. The oulet port must be connected to a component port that impose pressure.
      |
      | All parameters must be positive and eta0 must be in the [0 1] interval. the parameter cst_eff is boolean.
      mask init:
      | simscape.compiler.sli.internal.preinitmask(gcb);
      settings: CopyFcn=simscape.compiler.sli.internal.callback('CopyFcn',gcbh);  DeleteFcn=simscape.compiler.sli.internal.callback('DeleteFcn',gcbh);  ModelCloseFcn=simscape.compiler.sli.internal.callback('ModelCloseFcn',gcbh);  PreSaveFcn=simscape.compiler.sli.internal.callback('PreSaveFcn',gcbh);  PostSaveFcn=simscape.compiler.sli.internal.callback('PostSaveFcn',gcbh);  PreCopyFcn=simscape.compiler.sli.internal.callback('PreCopyFcn',gcbh);  PreDeleteFcn=simscape.compiler.sli.internal.callback('PreDeleteFcn',gcbh);
      mask Help: web(nesl_help(gcbh))
      mask TypeOptions A_conf: compiletime
      mask TypeOptions D_conf: compiletime
      mask TypeOptions Mass_conf: compiletime
      mask TypeOptions cst_eff_conf: compiletime | runtime
      mask TypeOptions eta0_conf: compiletime
      mask TypeOptions Tin0_conf: compiletime
      mask TypeOptions Pin0_conf: compiletime
      mask TypeOptions Pout0_conf: compiletime
      mask TypeOptions N0_conf: compiletime
      mask TypeOptions Q0_conf: compiletime
      mask TypeOptions v0_conf: compiletime
      mask TypeOptions I_conf: compiletime
      mask TypeOptions gamma_priority: None | Low | High
      mask TypeOptions C_priority: None | Low | High
      mask TypeOptions Z_priority: None | Low | High
      mask TypeOptions Cp_priority: None | Low | High
      mask TypeOptions Sin_priority: None | Low | High
      mask TypeOptions T_priority: None | Low | High
      mask TypeOptions HoutIs_priority: None | Low | High
      mask TypeOptions u1_priority: None | Low | High
      mask TypeOptions c1_priority: None | Low | High
      mask TypeOptions v_priority: None | Low | High
      mask TypeOptions eta_priority: None | Low | High
      mask TypeOptions eta_var_priority: None | Low | High
      mask TypeOptions N_priority: None | Low | High
      mask TypeOptions Q_priority: None | Low | High
      mask Display:
      | color('red');
      | port_label('RConn', 1,'out');
      | port_label('LConn', 1,'in');
  Turbine_p2 : SimscapeBlock  DialogController=NetworkEngine.DynNeDlgSource  LoadFcn=simscape.compiler.sli.internal.callback('LoadFcn',gcbh);  SourceFile=simCryogenics.Elements.Turbine_p2  mask(Turbine_p2){ComponentPath=simCryogenics.Elements.Turbine_p2, ComponentVariants=simCryogenics.Elements.Turbine_p2, ComponentVariantNames=Turbine_p2, ClassName=Turbine_p2, SchemaVersion=1, A=5e-6, A_unit=m^2, A_conf=compiletime, D=0.0255, D_unit=m, D_conf=compiletime, Mass=0.02, Mass_unit=kg, Mass_conf=compiletime, cst_eff=0, cst_eff_unit=1, cst_eff_conf=compiletime, eta0=0.8, eta0_unit=1, eta0_conf=compiletime, Tin0=20, Tin0_unit=K, Tin0_conf=compiletime, Pin0=16, Pin0_unit=bar, Pin0_conf=compiletime, Pout0=1.2, Pout0_unit=bar, Pout0_conf=compiletime, N0=2250, N0_unit=1/s, N0_conf=compiletime, Q0=0, Q0_unit=W, Q0_conf=compiletime, v0=0, v0_unit=1, v0_conf=compiletime, I=0, I_unit=kg*m^2, I_conf=compiletime, gamma_specify=off, gamma_priority=None, gamma=0, gamma_unit=1, C_specify=off, C_priority=None, C=0, C_unit=1, Z_specify=off, Z_priority=None, Z=0, Z_unit=1, Cp_specify=off, Cp_priority=None, Cp=0, Cp_unit=kJ/kg/K, Sin_specify=off, Sin_priority=None, Sin=0, Sin_unit=kJ/kg, T_specify=off, T_priority=None, T=0, T_unit=K, HoutIs_specify=off, HoutIs_priority=None, HoutIs=0, HoutIs_unit=kJ/kg, u1_specify=off, u1_priority=None, u1=0, u1_unit=m/s, c1_specify=off, c1_priority=None, c1=0, c1_unit=m/s, v_specify=off, v_priority=None, v=0, v_unit=1, eta_specify=off, eta_priority=None, eta=0, eta_unit=1, eta_var_specify=off, eta_var_priority=None, eta_var=0, eta_var_unit=1, N_specify=off, N_priority=None, N=0, N_unit=rad/s, Q_specify=off, Q_priority=None, Q=0, Q_unit=W, rp_crit_specify=off, rp_crit_priority=None, rp_crit=1, rp_crit_unit=1, rp_c_specify=off, rp_c_priority=None, rp_c=1, rp_c_unit=1}
      mask prompts: A "Section pass"; D "Blade diameter"; Mass "Shaft mass"; cst_eff "Constant efficiency"; eta0 "Nominal efficiency"; Tin0 "Nominal inlet temperature"; Pin0 "Nominal inlet pressure"; Pout0 "Nominal outlet pressure"; N0 "Nominal speed"; v0 "velocities ratio"; gamma_specify "gamma"; gamma_priority "gamma"; C_specify "C"; C_priority "C"; Z_specify "Z"; Z_priority "Z"; Cp_specify "Cp"; Cp_priority "Cp"; Sin_specify "Sin"; Sin_priority "Sin"; T_specify "T"; T_priority "T"; HoutIs_specify "HoutIs"; HoutIs_priority "HoutIs"; u1_specify "u1"; u1_priority "u1"; c1_specify "c1"; c1_priority "c1"; v_specify "v"; v_priority "v"; eta_specify "eta"; eta_priority "eta"; eta_var_specify "eta_var"; eta_var_priority "eta_var"; N_specify "N"; N_priority "N"; Q_specify "Q"; Q_priority "Q"; rp_crit_specify "rp_crit"; rp_crit_priority "rp_crit"; rp_c_specify "rp_c"; rp_c_priority "rp_c"
      mask help:
      | This component is a cryogenic Turbine with constant or variable isentropic efficiency. It impose the flowrate on both its inlet and oulet port. The outlet port also impose the temperature.
      |
      | To ensure compilation, this component inlet port must be connected to a component port that impose both temperature and pressure. The oulet port must be connected to a component port that impose pressure.
      |
      | All parameters must be positive and eta0 must be in the [0 1] interval. the parameter cst_eff is boolean.
      mask init:
      | simscape.compiler.sli.internal.preinitmask(gcb);
      settings: CopyFcn=simscape.compiler.sli.internal.callback('CopyFcn',gcbh);  DeleteFcn=simscape.compiler.sli.internal.callback('DeleteFcn',gcbh);  ModelCloseFcn=simscape.compiler.sli.internal.callback('ModelCloseFcn',gcbh);  PreSaveFcn=simscape.compiler.sli.internal.callback('PreSaveFcn',gcbh);  PostSaveFcn=simscape.compiler.sli.internal.callback('PostSaveFcn',gcbh);  PreCopyFcn=simscape.compiler.sli.internal.callback('PreCopyFcn',gcbh);  PreDeleteFcn=simscape.compiler.sli.internal.callback('PreDeleteFcn',gcbh);
      mask Help: web(nesl_help(gcbh))
      mask TypeOptions A_conf: compiletime
      mask TypeOptions D_conf: compiletime
      mask TypeOptions Mass_conf: compiletime
      mask TypeOptions cst_eff_conf: compiletime | runtime
      mask TypeOptions eta0_conf: compiletime
      mask TypeOptions Tin0_conf: compiletime
      mask TypeOptions Pin0_conf: compiletime
      mask TypeOptions Pout0_conf: compiletime
      mask TypeOptions N0_conf: compiletime
      mask TypeOptions Q0_conf: compiletime
      mask TypeOptions v0_conf: compiletime
      mask TypeOptions I_conf: compiletime
      mask TypeOptions gamma_priority: None | Low | High
      mask TypeOptions C_priority: None | Low | High
      mask TypeOptions Z_priority: None | Low | High
      mask TypeOptions Cp_priority: None | Low | High
      mask TypeOptions Sin_priority: None | Low | High
      mask TypeOptions T_priority: None | Low | High
      mask TypeOptions HoutIs_priority: None | Low | High
      mask TypeOptions u1_priority: None | Low | High
      mask TypeOptions c1_priority: None | Low | High
      mask TypeOptions v_priority: None | Low | High
      mask TypeOptions eta_priority: None | Low | High
      mask TypeOptions eta_var_priority: None | Low | High
      mask TypeOptions N_priority: None | Low | High
      mask TypeOptions Q_priority: None | Low | High
      mask TypeOptions rp_crit_priority: None | Low | High
      mask TypeOptions rp_c_priority: None | Low | High
      mask Display:
      | color('red');
      | port_label('RConn', 1,'out');
      | port_label('LConn', 1,'in');
  Valve : SimscapeBlock  DialogController=NetworkEngine.DynNeDlgSource  LoadFcn=simscape.compiler.sli.internal.callback('LoadFcn',gcbh);  SourceFile=simCryogenics.Elements.Valve  mask(Valve){ComponentPath=simCryogenics.Elements.Valve, ComponentVariants=simCryogenics.Elements.Valve, ComponentVariantNames=Valve, ClassName=Valve, SchemaVersion=1, CVmax=3.2, CVmax_unit=1, CVmax_conf=compiletime, ControlInputMin=0, ControlInputMin_unit=1, ControlInputMin_conf=compiletime, ControlInputMax=100, ControlInputMax_unit=1, ControlInputMax_conf=compiletime, Xt=0.86, Xt_unit=1, Xt_conf=compiletime, Rv=10, Rv_unit=1, Rv_conf=compiletime, lin_v=0, lin_v_unit=1, lin_v_conf=compiletime, lim_v=0, lim_v_unit=1, lim_v_conf=compiletime, K=2.4e-5, K_unit=m^1.50000*kg^0.50000/s/bar^0.50000, K_conf=compiletime, Cmd_specify=off, Cmd_priority=None, Cmd=0, Cmd_unit=1, gamma_specify=off, gamma_priority=None, gamma=0, gamma_unit=1, rho_specify=off, rho_priority=None, rho=0, rho_unit=kg/m^3, Xc_specify=off, Xc_priority=None, Xc=0, Xc_unit=1, X_specify=off, X_priority=None, X=0, X_unit=1, Y_specify=off, Y_priority=None, Y=0, Y_unit=1, CV_specify=off, CV_priority=None, CV=0, CV_unit=1}
      mask prompts: CVmax "Valve flow coefficient"; ControlInputMin "Minimum control input"; ControlInputMax "Maximum control output"; Xt "Xt valve constant"; Rv "Rv valve constant"; lin_v "Flow calculation method"; lim_v "Physical limit when treated as flowrate"; K "valve conversion factor"; Cmd_specify "Cmd"; Cmd_priority "Cmd"; gamma_specify "gamma"; gamma_priority "gamma"; rho_specify "rho"; rho_priority "rho"; Xc_specify "Xc"; Xc_priority "Xc"; X_specify "X"; X_priority "X"; Y_specify "Y"; Y_priority "Y"; CV_specify "CV"; CV_priority "CV"
      mask help:
      | This component is a valve.
      |
      | This model is imposing both flowrate end enthalpy on its outlet and floxrate on its inlet. The inlet port must be connected to a compent node that impose pressure and enthalpy. The oulet port must be connected to a coponent node that impose pressure
      |
      | All valve's parameters must be greather than 0
      mask init:
      | simscape.compiler.sli.internal.preinitmask(gcb);
      settings: CopyFcn=simscape.compiler.sli.internal.callback('CopyFcn',gcbh);  DeleteFcn=simscape.compiler.sli.internal.callback('DeleteFcn',gcbh);  ModelCloseFcn=simscape.compiler.sli.internal.callback('ModelCloseFcn',gcbh);  PreSaveFcn=simscape.compiler.sli.internal.callback('PreSaveFcn',gcbh);  PostSaveFcn=simscape.compiler.sli.internal.callback('PostSaveFcn',gcbh);  PreCopyFcn=simscape.compiler.sli.internal.callback('PreCopyFcn',gcbh);  PreDeleteFcn=simscape.compiler.sli.internal.callback('PreDeleteFcn',gcbh);
      mask Help: web(nesl_help(gcbh))
      mask TypeOptions CVmax_conf: compiletime
      mask TypeOptions ControlInputMin_conf: compiletime
      mask TypeOptions ControlInputMax_conf: compiletime
      mask TypeOptions Xt_conf: compiletime
      mask TypeOptions Rv_conf: compiletime
      mask TypeOptions lin_v_conf: compiletime | runtime
      mask TypeOptions lim_v_conf: compiletime | runtime
      mask TypeOptions K_conf: compiletime | runtime
      mask TypeOptions Cmd_priority: None | Low | High
      mask TypeOptions gamma_priority: None | Low | High
      mask TypeOptions rho_priority: None | Low | High
      mask TypeOptions Xc_priority: None | Low | High
      mask TypeOptions X_priority: None | Low | High
      mask TypeOptions Y_priority: None | Low | High
      mask TypeOptions CV_priority: None | Low | High
      mask Display:
      | color('red');
      | port_label('RConn', 1,'out');
      | port_label('LConn', 2,'in');
      | port_label('LConn', 1,'pos');
  Valve_ON_OFF : SimscapeBlock  DialogController=NetworkEngine.DynNeDlgSource  LoadFcn=simscape.compiler.sli.internal.callback('LoadFcn',gcbh);  SourceFile=simCryogenics.Elements.Valve_ON_OFF  mask(Valve_ON_OFF){ComponentPath=simCryogenics.Elements.Valve_ON_OFF, ComponentVariants=simCryogenics.Elements.Valve_ON_OFF, ComponentVariantNames=Valve_ON_OFF, ClassName=Valve_ON_OFF, SchemaVersion=1, CVmax=3.2, CVmax_unit=1, CVmax_conf=compiletime, ControlInputMin=0, ControlInputMin_unit=1, ControlInputMin_conf=compiletime, ControlInputMax=100, ControlInputMax_unit=1, ControlInputMax_conf=compiletime, Xt=0.86, Xt_unit=1, Xt_conf=compiletime, Rv=10, Rv_unit=1, Rv_conf=compiletime, lin_v=0, lin_v_unit=1, lin_v_conf=compiletime, lim_v=0, lim_v_unit=1, lim_v_conf=compiletime, K=2.4e-5, K_unit=m^1.50000*kg^0.50000/s/bar^0.50000, K_conf=compiletime, Cmd_specify=off, Cmd_priority=None, Cmd=0, Cmd_unit=1, gamma_specify=off, gamma_priority=None, gamma=0, gamma_unit=1, rho_specify=off, rho_priority=None, rho=0, rho_unit=kg/m^3, Xc_specify=off, Xc_priority=None, Xc=0, Xc_unit=1, X_specify=off, X_priority=None, X=0, X_unit=1, Y_specify=off, Y_priority=None, Y=0, Y_unit=1, CV_specify=off, CV_priority=None, CV=0, CV_unit=1}
      mask prompts: CVmax "Valve flow coefficient"; ControlInputMin "Minimum control input"; ControlInputMax "Maximum control output"; Xt "Xt valve constant"; Rv "Rv valve constant"; lin_v "Flow calculation method"; lim_v "Physical limit when treated as flowrate"; K "valve conversion factor"; Cmd_specify "Cmd"; Cmd_priority "Cmd"; gamma_specify "gamma"; gamma_priority "gamma"; rho_specify "rho"; rho_priority "rho"; Xc_specify "Xc"; Xc_priority "Xc"; X_specify "X"; X_priority "X"; Y_specify "Y"; Y_priority "Y"; CV_specify "CV"; CV_priority "CV"
      mask help:
      | This component is a ON/OFF valve. It impose the flow rate on both its inlet and outlet port. The outlet port also impose the temperature.
      |
      | To ensure compilation, the ON/OFF valve inlet port must be connected to a component  port that impose both temperature and pressure. The outlet port must be  connected to a component port that impose pressure.
      |
      | The parameters CVmax, Xt and Rv must be positive.
      mask init:
      | simscape.compiler.sli.internal.preinitmask(gcb);
      settings: CopyFcn=simscape.compiler.sli.internal.callback('CopyFcn',gcbh);  DeleteFcn=simscape.compiler.sli.internal.callback('DeleteFcn',gcbh);  ModelCloseFcn=simscape.compiler.sli.internal.callback('ModelCloseFcn',gcbh);  PreSaveFcn=simscape.compiler.sli.internal.callback('PreSaveFcn',gcbh);  PostSaveFcn=simscape.compiler.sli.internal.callback('PostSaveFcn',gcbh);  PreCopyFcn=simscape.compiler.sli.internal.callback('PreCopyFcn',gcbh);  PreDeleteFcn=simscape.compiler.sli.internal.callback('PreDeleteFcn',gcbh);
      mask Help: web(nesl_help(gcbh))
      mask TypeOptions CVmax_conf: compiletime
      mask TypeOptions ControlInputMin_conf: compiletime
      mask TypeOptions ControlInputMax_conf: compiletime
      mask TypeOptions Xt_conf: compiletime
      mask TypeOptions Rv_conf: compiletime
      mask TypeOptions lin_v_conf: compiletime | runtime
      mask TypeOptions lim_v_conf: compiletime | runtime
      mask TypeOptions K_conf: compiletime | runtime
      mask TypeOptions Cmd_priority: None | Low | High
      mask TypeOptions gamma_priority: None | Low | High
      mask TypeOptions rho_priority: None | Low | High
      mask TypeOptions Xc_priority: None | Low | High
      mask TypeOptions X_priority: None | Low | High
      mask TypeOptions Y_priority: None | Low | High
      mask TypeOptions CV_priority: None | Low | High
      mask Display:
      | color('red');
      | port_label('RConn', 1,'out');
      | port_label('LConn', 2,'in');
      | port_label('LConn', 1,'pos');
  inputQ : SimscapeBlock  DialogController=NetworkEngine.DynNeDlgSource  LoadFcn=simscape.compiler.sli.internal.callback('LoadFcn',gcbh);  SourceFile=simCryogenics.Elements.inputQ  mask(inputQ){ComponentPath=simCryogenics.Elements.inputQ, ComponentVariants=simCryogenics.Elements.inputQ, ComponentVariantNames=inputQ, ClassName=inputQ, SchemaVersion=1, N=1, N_unit=1, N_conf=compiletime}
      mask prompts: N "number of components"
      mask init:
      | simscape.compiler.sli.internal.preinitmask(gcb);
      settings: CopyFcn=simscape.compiler.sli.internal.callback('CopyFcn',gcbh);  DeleteFcn=simscape.compiler.sli.internal.callback('DeleteFcn',gcbh);  ModelCloseFcn=simscape.compiler.sli.internal.callback('ModelCloseFcn',gcbh);  PreSaveFcn=simscape.compiler.sli.internal.callback('PreSaveFcn',gcbh);  PostSaveFcn=simscape.compiler.sli.internal.callback('PostSaveFcn',gcbh);  PreCopyFcn=simscape.compiler.sli.internal.callback('PreCopyFcn',gcbh);  PreDeleteFcn=simscape.compiler.sli.internal.callback('PreDeleteFcn',gcbh);
      mask Help: web(nesl_help(gcbh))
      mask TypeOptions N_conf: compiletime | runtime
      mask Display:
      | disp('Simscape\n\n\n')
      | disp('\n\n\ninputQ');
      | color('red');
      | port_label('RConn', 1,'Qn');
      | port_label('LConn', 1,'Q1');
  isentropic : SimscapeBlock  DialogController=NetworkEngine.DynNeDlgSource  LoadFcn=simscape.compiler.sli.internal.callback('LoadFcn',gcbh);  SourceFile=simCryogenics.Elements.isentropic  mask(isentropic){ComponentPath=simCryogenics.Elements.isentropic, ComponentVariants=simCryogenics.Elements.isentropic, ComponentVariantNames=isentropic, ClassName=isentropic, SchemaVersion=1, eta=0.8, eta_unit=1, eta_conf=compiletime, Sin_specify=off, Sin_priority=None, Sin=0, Sin_unit=kJ/kg, HoutIs_specify=off, HoutIs_priority=None, HoutIs=0, HoutIs_unit=kJ/kg, Q_specify=off, Q_priority=None, Q=0, Q_unit=W}
      mask prompts: eta "Nominal efficiency"; Sin_specify "Sin"; Sin_priority "Sin"; HoutIs_specify "HoutIs"; HoutIs_priority "HoutIs"; Q_specify "Q"; Q_priority "Q"
      mask init:
      | simscape.compiler.sli.internal.preinitmask(gcb);
      settings: CopyFcn=simscape.compiler.sli.internal.callback('CopyFcn',gcbh);  DeleteFcn=simscape.compiler.sli.internal.callback('DeleteFcn',gcbh);  ModelCloseFcn=simscape.compiler.sli.internal.callback('ModelCloseFcn',gcbh);  PreSaveFcn=simscape.compiler.sli.internal.callback('PreSaveFcn',gcbh);  PostSaveFcn=simscape.compiler.sli.internal.callback('PostSaveFcn',gcbh);  PreCopyFcn=simscape.compiler.sli.internal.callback('PreCopyFcn',gcbh);  PreDeleteFcn=simscape.compiler.sli.internal.callback('PreDeleteFcn',gcbh);
      mask Help: web(nesl_help(gcbh))
      mask TypeOptions eta_conf: compiletime
      mask TypeOptions Sin_priority: None | Low | High
      mask TypeOptions HoutIs_priority: None | Low | High
      mask TypeOptions Q_priority: None | Low | High
      mask Display:
      | disp('Simscape\n\n\n')
      | disp('\n\n\nisentropic');
      | color('red');
      | port_label('LConn', 2,'Nominal efficiency');
      | port_label('RConn', 1,'out');
      | port_label('LConn', 1,'in');
  tuy_1D_3 : SimscapeBlock  DialogController=NetworkEngine.DynNeDlgSource  LoadFcn=simscape.compiler.sli.internal.callback('LoadFcn',gcbh);  SourceFile=simCryogenics.Elements.tuy_1D_3  mask(tuy_1D_3){ComponentPath=simCryogenics.Elements.tuy_1D_3, ComponentVariants=simCryogenics.Elements.tuy_1D_3, ComponentVariantNames=tuy_1D_3, ClassName=tuy_1D_3, SchemaVersion=1, V=1, V_unit=m^3, V_conf=compiletime, Pinit=10, Pinit_unit=bar, Pinit_conf=compiletime, Tinit=10, Tinit_unit=K, Tinit_conf=compiletime, K=1, K_unit=s*bar/kg, K_conf=compiletime, N=1, N_unit=1, N_conf=compiletime, Isochoric=0, Isochoric_unit=1, Isochoric_conf=compiletime}
      mask prompts: K "pressure loss coeficient"; N "number of control volume"; Isochoric "Isochoric 1/0"
      mask help:
      | It is composed with 20 tuyau_p_presion. It is a pipe that takes into account the pressure drop.
      |
      | Inlet port calculates incoming pressure and needs to be connected to an outlet that imposes flow rate and temperature.
      |
      | Outlet port imposes flow rate and enthalpy and must be connected to an intlet that imposes pressure.
      |
      | It has a heating input, where the heat is distributed between the number of activated inside tuyau.
      |
      | N states the number of working inside tuyau at a time.
      |
      | K is pressure loss coeffcient.
      |
      | It might work if the inlet pressure and temperature are imposed.
      mask init:
      | simscape.compiler.sli.internal.preinitmask(gcb);
      settings: CopyFcn=simscape.compiler.sli.internal.callback('CopyFcn',gcbh);  DeleteFcn=simscape.compiler.sli.internal.callback('DeleteFcn',gcbh);  ModelCloseFcn=simscape.compiler.sli.internal.callback('ModelCloseFcn',gcbh);  PreSaveFcn=simscape.compiler.sli.internal.callback('PreSaveFcn',gcbh);  PostSaveFcn=simscape.compiler.sli.internal.callback('PostSaveFcn',gcbh);  PreCopyFcn=simscape.compiler.sli.internal.callback('PreCopyFcn',gcbh);  PreDeleteFcn=simscape.compiler.sli.internal.callback('PreDeleteFcn',gcbh);
      mask Help: web(nesl_help(gcbh))
      mask TypeOptions V_conf: compiletime | runtime
      mask TypeOptions Pinit_conf: compiletime
      mask TypeOptions Tinit_conf: compiletime
      mask TypeOptions K_conf: compiletime | runtime
      mask TypeOptions N_conf: compiletime | runtime
      mask TypeOptions Isochoric_conf: compiletime | runtime
      mask Display:
      | disp('Simscape\n\n\n')
      | disp('\n\n\ntuy_1D_3');
      | color('red');
      | port_label('LConn', 2,'');
      | port_label('RConn', 1,'');
      | port_label('LConn', 1,'');
  tuyau_p.presion : SimscapeBlock  DialogController=NetworkEngine.DynNeDlgSource  LoadFcn=simscape.compiler.sli.internal.callback('LoadFcn',gcbh);  SourceFile=simCryogenics.Elements.tuyau_p_presion  mask(tuyau_p.presion){ComponentPath=simCryogenics.Elements.tuyau_p_presion, ComponentVariants=simCryogenics.Elements.tuyau_p_presion, ComponentVariantNames=tuyau_p_presion, ClassName=tuyau_p_presion, SchemaVersion=1, V=0, V_unit=m^3, V_conf=compiletime, Pinit=10, Pinit_unit=bar, Pinit_conf=compiletime, Tinit=10, Tinit_unit=K, Tinit_conf=compiletime, K=0, K_unit=s*bar/kg, K_conf=compiletime, act=1, act_unit=1, act_conf=compiletime, Isochoric=0, Isochoric_unit=1, Isochoric_conf=compiletime, rho_specify=off, rho_priority=None, rho=10, rho_unit=kg/m^3, u_specify=off, u_priority=None, u=1000, u_unit=J/kg}
      mask prompts: Isochoric "Isochoric 1/0"; rho_specify "rho"; rho_priority "rho"; u_specify "u"; u_priority "u"
      mask init:
      | simscape.compiler.sli.internal.preinitmask(gcb);
      settings: CopyFcn=simscape.compiler.sli.internal.callback('CopyFcn',gcbh);  DeleteFcn=simscape.compiler.sli.internal.callback('DeleteFcn',gcbh);  ModelCloseFcn=simscape.compiler.sli.internal.callback('ModelCloseFcn',gcbh);  PreSaveFcn=simscape.compiler.sli.internal.callback('PreSaveFcn',gcbh);  PostSaveFcn=simscape.compiler.sli.internal.callback('PostSaveFcn',gcbh);  PreCopyFcn=simscape.compiler.sli.internal.callback('PreCopyFcn',gcbh);  PreDeleteFcn=simscape.compiler.sli.internal.callback('PreDeleteFcn',gcbh);
      mask Help: web(nesl_help(gcbh))
      mask TypeOptions V_conf: compiletime | runtime
      mask TypeOptions Pinit_conf: compiletime
      mask TypeOptions Tinit_conf: compiletime
      mask TypeOptions K_conf: compiletime | runtime
      mask TypeOptions act_conf: compiletime | runtime
      mask TypeOptions Isochoric_conf: compiletime
      mask TypeOptions rho_priority: None | Low | High
      mask TypeOptions u_priority: None | Low | High
      mask Display:
      | disp('Simscape\n\n\n')
      | disp('\n\n\ntuyau_p_presion');
      | color('red');
      | port_label('LConn', 2,'');
      | port_label('RConn', 1,'');
      | port_label('LConn', 1,'');
